simulink model "EXPERIMENT_06"  (R2023b)
settings: Solver=VariableStepAuto  StartTime=0.0  StopTime=20  RelTol=1e-3
libraries: spsDCVoltageSourceLib x2, spsDCMachineLib x1, sps_lib x1
settings Model: Creator=deves  LastModifiedBy=deves

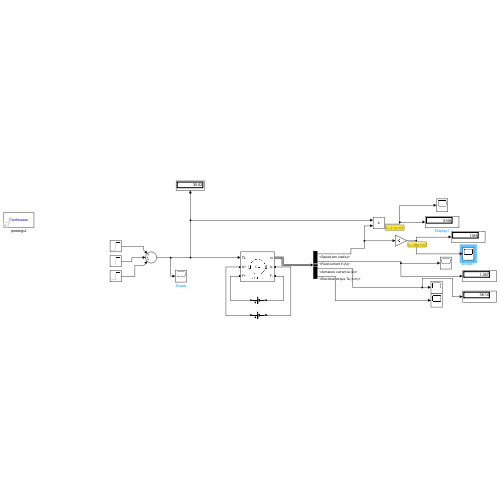
[thumbnail: Simulink's stored preview of the top-level diagram]
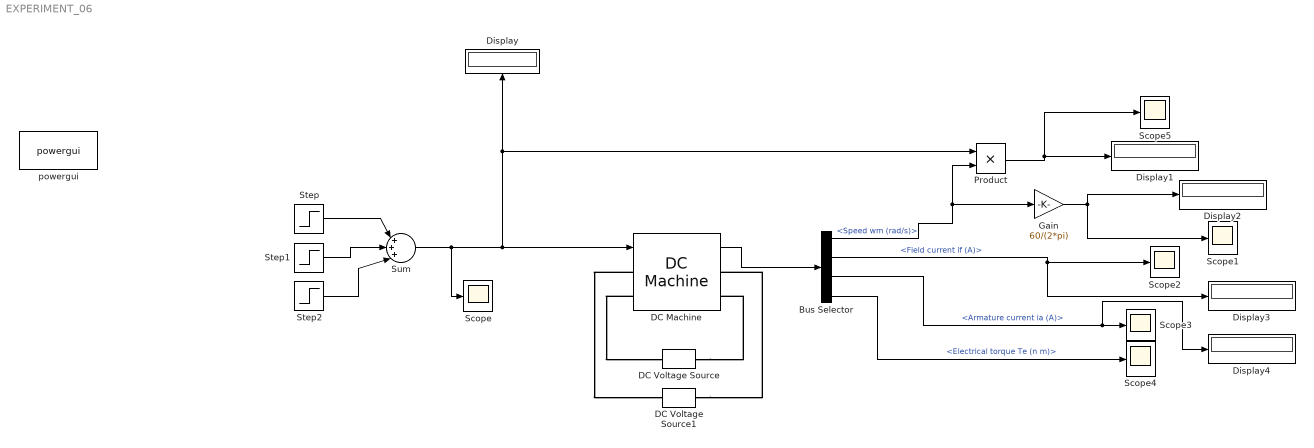
== system EXPERIMENT_06 ==
  Bus Selector : BusSelector  OutputSignals=Speed wm (rad/s),Field current if (A),Armature current ia (A),Electrical torque Te (n m)
  DC Machine : spsDCMachineLib/DC Machine  PresetModel=01: 5HP 240V 1750RPM Field:300V  MechanicalLoad=Torque TL  FieldType=Wound  ShowDetailedParameters=on  MeasurementBus=off  RLa=[2.581 0.028]  RLf=[281.2 156]  Laf=0.9483  MachineConstant=Torque constant (N.m/A)  Ke=1.8  Kt=1.8  J=0.02215  Bm=0.002953  Tf=0.5161  w0=1  Ifinit=1.06685633001422  TsPowergui=0  TsBlock=-1
  DC Voltage Source : spsDCVoltageSourceLib/DC Voltage Source  Amplitude=300  Measurements=None
  DC Voltage Source1 : spsDCVoltageSourceLib/DC Voltage Source  Amplitude=240  Measurements=None
  Display{,1..4} (5 alike) : Display
  Gain : Gain  Gain=60/(2*pi)
  Product : Product
  Scope{,1..5} (6 alike) : Scope
  Step : Step  After=20.353 * 0.25  SampleTime=0
  Step1 : Step  Time=2  After=20.353*0.5  SampleTime=0
  Step2 : Step  Time=3  After=20.353  SampleTime=0
  Sum : Sum  Inputs=|+++|
  powergui : sps_lib/powergui  Priority=1  SimulationMode=Continuous  SampleTime=50e-6  frequency=60  Iterations=50  frequencyindice=0  Pbase=100e6  ErrMax=1e-4  UnitsV=kV  UnitsW=MW  buscounter=0  FunctionMessages=off  echomessages=off  EnableUseOfTLC=off  CurrentSourceSwitches=off  DisableSnubberDevices=off  DisableRonSwitches=off  DisableVfSwitches=off  DisplayEquations=off  AutomaticDiscreteSolvers=off  SolverType=Tustin/Backward Euler (TBE)  Interpol=off  ExternalGateDelay=off  methode=off  Ts=100  x0status=blocks  SPID=on  SwTol=0  HookPort=off  NonlinearTolerance=1e-4  nMaxIteration=100  ContinueOnMaxIteration=off  RestoreLinks=warning  ResistiveCurrentMeasurement=off  Frange=[0:2:500]  Ylog=off  Xlog=on  ShowGrid=off  save=off  variable=ZData  structure=0  ZoomFFT=off  StartTime=0.0  cycles=1  DisplayStyle=1  fundamental=60  FreqAxis=off  MaxFrequency=1000  frequencyindicesteady=1  RmsSteady=1  display=off
  wires:
  Step/1 -> Sum/1
  Step1/1 -> Sum/2
  Step2/1 -> Sum/3
  Sum/1 -> Scope/1, DC Machine/1, Display/1, Product/1
  Bus Selector/2 -> Display3/1, Scope2/1  "<Field current if (A)>"
  DC Machine/1 -> Bus Selector/1
  Bus Selector/4 -> Scope4/1  "<Electrical torque Te (n m)>"
  Bus Selector/3 -> Display4/1, Scope3/1  "<Armature current ia (A)>"
  Bus Selector/1 -> Gain/1, Product/2  "<Speed wm (rad/s)>"
  Product/1 -> Scope5/1, Display1/1
  Gain/1 -> Scope1/1, Display2/1
  connections:
  DC Machine/LConn2 -- DC Voltage Source/RConn1
  DC Machine/LConn1 -- DC Voltage Source1/RConn1
  DC Voltage Source1/LConn1 -- DC Machine/RConn1
  DC Voltage Source/LConn1 -- DC Machine/RConn2
